simulink model "AFDNFSmodelSPA"  (R2017b)
settings: Solver=ode45  StartTime=0.0  StopTime=1400  FixedStep=1e-3  RelTol=1e-8  EnableMultiTasking=on
PostLoadFcn:
  | run('Methods/NFSOnLoad');
InitFcn:
  | run('Methods/AFDSimInit')
StopFcn:
  | run('Methods/NFSOnLoad');
values from neighbouring files (symbols this model uses):
  nfs = TransferFunction('Plot','true')    [Main.m]    (also in NFSDatabase.sldd = SI
                Imperial
                28184.4409185639)
undefined symbols (not defined in the file or in its folder): Continuous, desired, Earth, F, K_lat, K_long, Kobsvlat, Kobsvlong, lat, latsys, Light, long, longsys, MIL, Newton, Raphson, sigbuilder_block, Time, WGS84
libraries: simulink x6, aerolibtransform2 x2, aerolibwind2 x2, ModelsLibrary x1, ctrlSharedLib x1, sharedutil x1
(part 3 of 4)

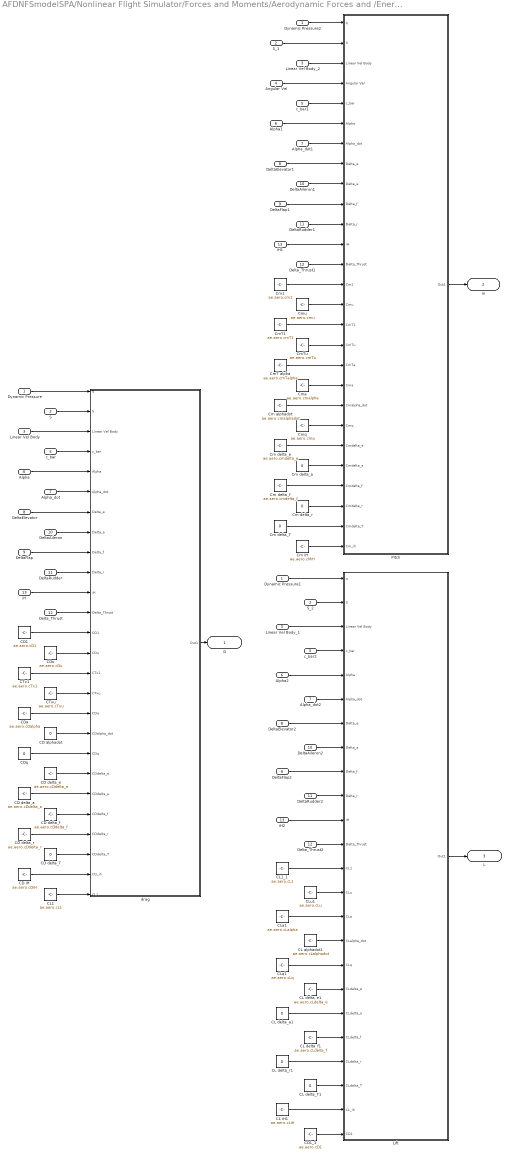
== system AFDNFSmodelSPA/Nonlinear Flight Simulator/Forces and Moments/Aerodynamic Forces and /Energy Analysis1/Longitudinal1 ==
  Dynamic Pressure : Inport
  S : Inport  Port=2
  Linear Vel Body : Inport  Port=3
  Angular Vel : Inport  Port=4
  c_bar : Inport  Port=5
  Alpha : Inport  Port=6
  Alpha_dot : Inport  Port=7
  DeltaElevator : Inport  Port=8
  DeltaFlap : Inport  Port=9
  DeltaAileron : Inport  Port=10
  DeltaRudder : Inport  Port=11
  Delta_Thrust : Inport  Port=12
  iH : Inport  Port=13
  Alpha1 : InportShadow  Port=6
  Alpha2 : InportShadow  Port=6
  Alpha_dot1 : InportShadow  Port=7
  Alpha_dot2 : InportShadow  Port=7
  CD alphadot : Constant  Value=0
  CD delta_T : Constant  Value=0
  CD delta_a : Constant  Value=ae.aero.cDdelta_a
  CD delta_e : Constant  Value=ae.aero.cDdelta_e
  CD delta_f : Constant  Value=ae.aero.cDdelta_f
  CD delta_r : Constant  Value=ae.aero.cDdelta_r
  CD iH : Constant  Value=ae.aero.cDiH
  CD1 : Constant  Value=ae.aero.cD1
  CD1_1 : Constant  Value=ae.aero.cD1
  CDa : Constant  Value=ae.aero.cDalpha
  CDq : Constant  Value=0
  CDu : Constant  Value=ae.aero.cDu
  CL alphadot1 : Constant  Value=ae.aero.cLalphadot
  CL delta_T1 : Constant  Value=0
  CL delta_a1 : Constant  Value=0
  CL delta_e1 : Constant  Value=ae.aero.cLdelta_e
  CL delta_f1 : Constant  Value=ae.aero.cLdelta_f
  CL delta_r1 : Constant  Value=0
  CL iH1 : Constant  Value=ae.aero.cLiH
  CL1 : Constant  Value=ae.aero.cL1
  CL1_1 : Constant  Value=ae.aero.cL1
  CLa1 : Constant  Value=ae.aero.cLalpha
  CLq1 : Constant  Value=ae.aero.cLq
  CLu1 : Constant  Value=ae.aero.cLu
  CTx1 : Constant  Value=ae.aero.cTx1
  CTxu : Constant  Value=ae.aero.cTxu
  Cm alphadot : Constant  Value=ae.aero.cmalphadot
  Cm delta_T : Constant  Value=0
  Cm delta_a : Constant  Value=0
  Cm delta_e : Constant  Value=ae.aero.cmdelta_e
  Cm delta_f : Constant  Value=ae.aero.cmdelta_f
  Cm delta_r : Constant  Value=0
  Cm iH : Constant  Value=ae.aero.cMiH
  Cm1 : Constant  Value=ae.aero.cm1
  CmT alpha : Constant  Value=ae.aero.cmTalpha
  CmT1 : Constant  Value=ae.aero.cmT1
  CmTu : Constant  Value=ae.aero.cmTu
  Cma : Constant  Value=ae.aero.cmalpha
  Cmq : Constant  Value=ae.aero.cmq
  Cmu : Constant  Value=ae.aero.cmu
  DeltaAileron1 : InportShadow  Port=10
  DeltaAileron2 : InportShadow  Port=10
  DeltaElevator1 : InportShadow  Port=8
  DeltaElevator2 : InportShadow  Port=8
  DeltaFlap1 : InportShadow  Port=9
  DeltaFlap2 : InportShadow  Port=9
  DeltaRudder1 : InportShadow  Port=11
  DeltaRudder2 : InportShadow  Port=11
  Delta_Thrust1 : InportShadow  Port=12
  Delta_Thrust2 : InportShadow  Port=12
  Dynamic Pressure1 : InportShadow
  Dynamic Pressure2 : InportShadow
  Lift : Subsystem
  Linear Vel Body_1 : InportShadow  Port=3
  Linear Vel Body_2 : InportShadow  Port=3
  Pitch : Subsystem
  S_1 : InportShadow  Port=2
  S_2 : InportShadow  Port=2
  c_bar1 : InportShadow  Port=5
  c_bar2 : InportShadow  Port=5
  drag : Subsystem
  iH1 : InportShadow  Port=13
  iH2 : InportShadow  Port=13
  D : Outport
  m : Outport  Port=2
  L : Outport  Port=3
  wires:
  DeltaRudder/1 -> drag/10(Delta_r)
  DeltaAileron/1 -> drag/8(Delta_a)
  CDa/1 -> drag/17(CDa)
  Alpha/1 -> drag/5(Alpha)
  CDu/1 -> drag/14(CDu)
  Alpha_dot/1 -> drag/6(Alpha_dot)
  drag/1(Out1) -> D/1
  Lift/1(Out1) -> L/1
  S/1 -> drag/2(S)
  Dynamic Pressure/1 -> drag/1(q)
  Linear Vel Body/1 -> drag/3(Linear Vel Body)
  Delta_Thrust/1 -> drag/12(Delta_Thrust)
  iH/1 -> drag/11(iH)
  CD delta_T/1 -> drag/24(CDdelta_T)
  DeltaElevator/1 -> drag/7(Delta_e)
  DeltaFlap/1 -> drag/9(Delta_f)
  Pitch/1(Out1) -> m/1
  c_bar/1 -> drag/4(c_bar)
  CD alphadot/1 -> drag/18(CDalpha_dot)
  CDq/1 -> drag/19(CDq)
  CD delta_e/1 -> drag/20(CDdelta_e)
  CD delta_a/1 -> drag/21(CDdelta_a)
  CD delta_f/1 -> drag/22(CDdelta_f)
  CD delta_r/1 -> drag/23(CDdelta_r)
  CD iH/1 -> drag/25(CD_ih)
  CTx1/1 -> drag/15(CTx1)
  CD1/1 -> drag/13(CD1)
  CTxu/1 -> drag/16(CTxu)
  DeltaRudder1/1 -> Pitch/11(Delta_r)
  DeltaAileron1/1 -> Pitch/9(Delta_a)
  Alpha1/1 -> Pitch/6(Alpha)
  Alpha_dot1/1 -> Pitch/7(Alpha_dot)
  S_1/1 -> Pitch/2(S)
  Dynamic Pressure2/1 -> Pitch/1(q)
  Linear Vel Body_2/1 -> Pitch/3(Linear Vel Body)
  Delta_Thrust1/1 -> Pitch/13(Delta_Thrust)
  iH1/1 -> Pitch/12(iH)
  DeltaElevator1/1 -> Pitch/8(Delta_e)
  DeltaFlap1/1 -> Pitch/10(Delta_f)
  S_2/1 -> Lift/2(S)
  Dynamic Pressure1/1 -> Lift/1(q)
  Linear Vel Body_1/1 -> Lift/3(Linear Vel Body)
  Delta_Thrust2/1 -> Lift/12(Delta_Thrust)
  c_bar2/1 -> Lift/4(c_bar)
  CL1/1 -> drag/26(CL1)
  iH2/1 -> Lift/11(iH)
  DeltaRudder2/1 -> Lift/10(Delta_r)
  DeltaFlap2/1 -> Lift/9(Delta_f)
  DeltaAileron2/1 -> Lift/8(Delta_a)
  DeltaElevator2/1 -> Lift/7(Delta_e)
  Alpha_dot2/1 -> Lift/6(Alpha_dot)
  Alpha2/1 -> Lift/5(Alpha)
  Angular Vel/1 -> Pitch/4(Angular Vel)
  c_bar1/1 -> Pitch/5(c_bar)
  CD1_1/1 -> Lift/24(CD1)
  CLa1/1 -> Lift/15(CLa)
  CLq1/1 -> Lift/17(CLq)
  CL delta_a1/1 -> Lift/19(CLdelta_a)
  CL delta_r1/1 -> Lift/21(CLdelta_r)
  CL iH1/1 -> Lift/23(CL_ih)
  CL delta_T1/1 -> Lift/22(CLdelta_T)
  CLu1/1 -> Lift/14(CLu)
  CL alphadot1/1 -> Lift/16(CLalpha_dot)
  CL delta_f1/1 -> Lift/20(CLdelta_f)
  CL delta_e1/1 -> Lift/18(CLdelta_e)
  CL1_1/1 -> Lift/13(CL1)
  CmT alpha/1 -> Pitch/18(CmTa)
  Cm alphadot/1 -> Pitch/20(Cmalpha_dot)
  Cm delta_e/1 -> Pitch/22(Cmdelta_e)
  Cm delta_f/1 -> Pitch/24(Cmdelta_f)
  Cm delta_T/1 -> Pitch/26(Cmdelta_T)
  CmT1/1 -> Pitch/16(CmT1)
  Cm1/1 -> Pitch/14(Cm1)
  CmTu/1 -> Pitch/17(CmTu)
  Cmq/1 -> Pitch/21(Cmq)
  Cm delta_a/1 -> Pitch/23(Cmdelta_a)
  Cm delta_r/1 -> Pitch/25(Cmdelta_r)
  Cmu/1 -> Pitch/15(Cmu)
  Cma/1 -> Pitch/19(Cma)
  Cm iH/1 -> Pitch/27(Cm_ih)

== system AFDNFSmodelSPA/Nonlinear Flight Simulator/Forces and Moments/Aerodynamic Forces and /Forces/Aerodynamic Forces ==
  note: Since the forces and moments are in stability axis,
      | the beta has been multiplied with zero.
  CL : Inport  PortDimensions=1
  CD : Inport  Port=2  PortDimensions=1
  CY : Inport  Port=3  PortDimensions=1
  Dynamic Pressure : Inport  Port=4  PortDimensions=1
  Alpha : Inport  Port=5  PortDimensions=1
  Beta : Inport  Port=6  PortDimensions=1
  ChSign : Gain  Gain=-1  SaturateOnIntegerOverflow=on  OutDataTypeStr=Inherit: Same as input  ParamDataTypeStr=Inherit: Same as input
  ChSign1 : Gain  Gain=-1  SaturateOnIntegerOverflow=on  OutDataTypeStr=Inherit: Same as input  ParamDataTypeStr=Inherit: Same as input
  ChSign2 : Gain  Gain=0  SaturateOnIntegerOverflow=on  OutDataTypeStr=Inherit: Same as input  ParamDataTypeStr=Inherit: Same as input
  Mux : Mux  Inputs=3
  Product{,2..4} (4 alike) : Product  SaturateOnIntegerOverflow=on  InputSameDT=on  OutDataTypeStr=Inherit: Same as first input
  Product1 : Product  Multiplication=Matrix(*)  SaturateOnIntegerOverflow=on  InputSameDT=on  OutDataTypeStr=Inherit: Same as first input
  Wind2Body TM : Subsystem
  Wing Area : Constant  Value=nfs.refarea
  Aerodynamic Forces : Outport  PortDimensions=[3,1]
  wires:
  Wind2Body TM/1(T_BW) -> Product1/1
  Product1/1 -> Aerodynamic Forces/1
  Beta/1 -> ChSign2/1
  CD/1 -> ChSign/1
  CL/1 -> ChSign1/1
  Alpha/1 -> Wind2Body TM/1(Alpha)
  Dynamic Pressure/1 -> Product/1
  Wing Area/1 -> Product/2
  Product/1 -> Product2/1, Product3/1, Product4/1
  ChSign/1 -> Product2/2
  CY/1 -> Product3/2
  ChSign1/1 -> Product4/2
  Product2/1 -> Mux/1
  Product3/1 -> Mux/2
  Product4/1 -> Mux/3
  Mux/1 -> Product1/2
  ChSign2/1 -> Wind2Body TM/2(Beta)

== system AFDNFSmodelSPA/Nonlinear Flight Simulator/Forces and Moments/Aerodynamic Forces and /Forces/Force Coefficients Calculator ==
  Linear Velocity : Inport  PortDimensions=[3,1]
  Alpha : Inport  Port=2  PortDimensions=1
  Beta : Inport  Port=3
  Angular Velocity : Inport  Port=4  PortDimensions=[3,1]
  Control : Inport  Port=5  PortDimensions=[4,1]
  Alphadot : Inport  Port=6  PortDimensions=1
  Mach : Inport  Port=7
  Alpha2 : InportShadow  Port=2  PortDimensions=1
  Angular Velocity1 : InportShadow  Port=4  PortDimensions=[3,1]
  Control1 : InportShadow  Port=5  PortDimensions=[4,1]
  Demux1 : Demux  Outputs=3
  Demux2 : Demux  Outputs=3
  Demux3 : Demux
  Demux4 : Demux
  Drag Coefficient : Subsystem  mask{cD0=nfs.aero.cD0}
  Lift Coefficient : Subsystem  mask{cL0=nfs.aero.cL0, meanchord=nfs.meanchord}
      mask prompts: meanchord "Mean Aerodynamic Chord"
  Linear Velocity1 : InportShadow  PortDimensions=[3,1]
  Mach1 : InportShadow  Port=7
  SideForce Coefficient : Subsystem
  Terminator{,1..4} (5 alike) : Terminator
  CL : Outport
  CD : Outport  Port=2
  CY : Outport  Port=3
  wires:
  Linear Velocity/1 -> Lift Coefficient/1(Linear Velocity)
  SideForce Coefficient/1(CY) -> CY/1
  Drag Coefficient/1(CD) -> CD/1
  Alpha2/1 -> Drag Coefficient/2(alpha)
  Demux1/3 -> Terminator1/1
  Alphadot/1 -> Lift Coefficient/5(Alphadot)
  Lift Coefficient/1(CL) -> CL/1, Drag Coefficient/1(CL)
  Demux2/1 -> SideForce Coefficient/3(P)
  Demux3/1 -> Lift Coefficient/3(DeltaElevator)
  Control1/1 -> Demux4/1
  Demux2/3 -> SideForce Coefficient/4(R)
  Angular Velocity1/1 -> Demux2/1
  Beta/1 -> SideForce Coefficient/2(Beta)
  Demux1/1 -> Terminator/1
  Control/1 -> Demux3/1
  Angular Velocity/1 -> Demux1/1
  Demux4/2 -> Drag Coefficient/4(DeltaFlap)
  Mach/1 -> Lift Coefficient/7(Mach)
  Demux1/2 -> Lift Coefficient/6(Q)
  Demux3/4 -> Terminator4/1
  Demux3/3 -> Terminator3/1
  Alpha/1 -> Lift Coefficient/2(Alpha)
  Demux2/2 -> Terminator2/1
  Demux4/4 -> SideForce Coefficient/6(DeltaRudder), Drag Coefficient/6(DeltaRudder)
  Demux4/3 -> SideForce Coefficient/5(DeltaAileron), Drag Coefficient/5(DeltaAileron)
  Demux4/1 -> Drag Coefficient/3(DeltaElevator)
  Mach1/1 -> Drag Coefficient/7(Mach)
  Demux3/2 -> Lift Coefficient/4(DeltaFlap)
  Linear Velocity1/1 -> SideForce Coefficient/1(Linear Velocity)

== system AFDNFSmodelSPA/Nonlinear Flight Simulator/Forces and Moments/Aerodynamic Forces and /Moments/Aerodynamic Moment  ==
  note: Since the forces and moments are in stability axis,
      | the beta has been multiplied with zero.
  Cl : Inport
  Cm : Inport  Port=2
  Cn : Inport  Port=3
  Dynamic Pressure : Inport  Port=4
  Alpha : Inport  Port=5  PortDimensions=1
  Beta : Inport  Port=6  PortDimensions=1
  Dynamic Pressure1 : InportShadow  Port=4
  Dynamic Pressure2 : InportShadow  Port=4
  Gain : Gain  Gain=0
  Mux : Mux  Inputs=3
  Pitch : Product  Inputs=4  SaturateOnIntegerOverflow=on  InputSameDT=on  OutDataTypeStr=Inherit: Same as first input
  Product1 : Product  Multiplication=Matrix(*)  SaturateOnIntegerOverflow=on  InputSameDT=on  OutDataTypeStr=Inherit: Same as first input
  Roll : Product  Inputs=4  SaturateOnIntegerOverflow=on  InputSameDT=on  OutDataTypeStr=Inherit: Same as first input
  Wind2Body TM : Subsystem
  Wing area : Constant  Value=nfs.refarea
  Wing chord : Constant  Value=nfs.meanchord
  Wing span : Constant  Value=nfs.span
  Wing span2 : Constant  Value=nfs.span
  Yaw : Product  Inputs=4  SaturateOnIntegerOverflow=on  InputSameDT=on  OutDataTypeStr=Inherit: Same as first input
  Aerodynamic Moments : Outport  PortDimensions=[3,1]
  wires:
  Yaw/1 -> Mux/3
  Pitch/1 -> Mux/2
  Roll/1 -> Mux/1
  Wing area/1 -> Yaw/2, Roll/2, Pitch/2
  Wing span2/1 -> Yaw/3
  Dynamic Pressure2/1 -> Yaw/1
  Dynamic Pressure1/1 -> Pitch/1
  Cl/1 -> Roll/4
  Cm/1 -> Pitch/4
  Cn/1 -> Yaw/4
  Dynamic Pressure/1 -> Roll/1
  Wing chord/1 -> Pitch/3
  Wing span/1 -> Roll/3
  Wind2Body TM/1(T_BW) -> Product1/1
  Beta/1 -> Gain/1
  Alpha/1 -> Wind2Body TM/1(Alpha)
  Mux/1 -> Product1/2
  Product1/1 -> Aerodynamic Moments/1
  Gain/1 -> Wind2Body TM/2(Beta)

== system AFDNFSmodelSPA/Nonlinear Flight Simulator/Forces and Moments/Aerodynamic Forces and /Moments/Pitch Moment Coefficient ==
  Linear Velocity : Inport
  Alpha : Inport  Port=2
  Q : Inport  Port=3
  DeltaElevator : Inport  Port=4
  DeltaFlap : Inport  Port=5
  Alphadot : Inport  Port=6  PortDimensions=1
  Mach : Inport  Port=7  PortDimensions=1
  2 : Gain  Gain=2  SaturateOnIntegerOverflow=on  OutDataTypeStr=Inherit: Same as input  ParamDataTypeStr=Inherit: Same as input
  Cm*c/(2V) : Product  Inputs=**/  SaturateOnIntegerOverflow=on  InputSameDT=on  OutDataTypeStr=Inherit: Same as first input
  Cm0 : Constant  Value=nfs.aero.cm0
  Scope{1..7} (7 alike) : Scope
  Sum : Sum  SaturateOnIntegerOverflow=on  InputSameDT=on  OutDataTypeStr=Inherit: Same as first input
  Sum2 : Sum  Inputs=++++++  SaturateOnIntegerOverflow=on  InputSameDT=on  OutDataTypeStr=Inherit: Same as first input
  Velocity Magnitude : Subsystem
  Wing chord : Constant  Value=nfs.meanchord
  cmM : Gain  Gain=nfs.aero.cmM  SaturateOnIntegerOverflow=on  OutDataTypeStr=Inherit: Same as input  ParamDataTypeStr=Inherit: Same as input
  cmalpha : Gain  Gain=nfs.aero.cmalpha  SaturateOnIntegerOverflow=on  OutDataTypeStr=Inherit: Same as input  ParamDataTypeStr=Inherit: Same as input
  cmalphadot : Gain  Gain=nfs.aero.cmalphadot  SaturateOnIntegerOverflow=on  OutDataTypeStr=Inherit: Same as input  ParamDataTypeStr=Inherit: Same as input
  cmdelta_e : Gain  Gain=nfs.aero.cmdelta_e  SaturateOnIntegerOverflow=on  OutDataTypeStr=Inherit: Same as input  ParamDataTypeStr=Inherit: Same as input
  cmdelta_f : Gain  Gain=nfs.aero.cmdelta_f  SaturateOnIntegerOverflow=on  OutDataTypeStr=Inherit: Same as input  ParamDataTypeStr=Inherit: Same as input
  cmq : Gain  Gain=nfs.aero.cmq  SaturateOnIntegerOverflow=on  OutDataTypeStr=Inherit: Same as input  ParamDataTypeStr=Inherit: Same as input
  Cm : Outport  PortDimensions=1
  wires:
  Sum2/1 -> Cm/1
  Mach/1 -> cmM/1
  Q/1 -> cmq/1
  DeltaElevator/1 -> cmdelta_e/1
  DeltaFlap/1 -> cmdelta_f/1
  Alpha/1 -> cmalpha/1
  Velocity Magnitude/1(Velocity Magnitude) -> 2/1
  Linear Velocity/1 -> Velocity Magnitude/1(Velocity)
  cmM/1 -> Sum2/6, Scope6/1
  Cm*c/(2V)/1 -> Sum2/5
  cmdelta_e/1 -> Sum2/4, Scope3/1
  cmdelta_f/1 -> Sum2/3, Scope2/1
  cmalpha/1 -> Sum2/2, Scope1/1
  Cm0/1 -> Sum2/1, Scope7/1
  Sum/1 -> Cm*c/(2V)/1
  cmalphadot/1 -> Sum/1, Scope4/1
  cmq/1 -> Sum/2, Scope5/1
  Wing chord/1 -> Cm*c/(2V)/2
  2/1 -> Cm*c/(2V)/3
  Alphadot/1 -> cmalphadot/1

== system AFDNFSmodelSPA/Nonlinear Flight Simulator/Forces and Moments/Aerodynamic Forces and /Moments/Roll Moment Coefficient ==
  Linear Velocity : Inport
  Beta : Inport  Port=2  PortDimensions=1
  P : Inport  Port=3
  R : Inport  Port=4
  DeltaAileron : Inport  Port=5
  DeltaRudder : Inport  Port=6
  2 : Gain  Gain=2  SaturateOnIntegerOverflow=on  OutDataTypeStr=Inherit: Same as input  ParamDataTypeStr=Inherit: Same as input
  Cl*b/(2V) : Product  Inputs=**/  SaturateOnIntegerOverflow=on  InputSameDT=on  OutDataTypeStr=Inherit: Same as first input
  Sum : Sum  SaturateOnIntegerOverflow=on  InputSameDT=on  OutDataTypeStr=Inherit: Same as first input
  Sum2 : Sum  Inputs=++++  SaturateOnIntegerOverflow=on  InputSameDT=on  OutDataTypeStr=Inherit: Same as first input
  Velocity Magnitude : Subsystem
  Wing span : Constant  Value=nfs.span
  clbeta : Gain  Gain=nfs.aero.clbeta  SaturateOnIntegerOverflow=on  OutDataTypeStr=Inherit: Same as input  ParamDataTypeStr=Inherit: Same as input
  cldelta_a : Gain  Gain=nfs.aero.cldelta_a  SaturateOnIntegerOverflow=on  OutDataTypeStr=Inherit: Same as input  ParamDataTypeStr=Inherit: Same as input
  cldelta_r : Gain  Gain=nfs.aero.cldelta_r  SaturateOnIntegerOverflow=on  OutDataTypeStr=Inherit: Same as input  ParamDataTypeStr=Inherit: Same as input
  clp : Gain  Gain=nfs.aero.clp  SaturateOnIntegerOverflow=on  OutDataTypeStr=Inherit: Same as input  ParamDataTypeStr=Inherit: Same as input
  clr : Gain  Gain=nfs.aero.clr  SaturateOnIntegerOverflow=on  OutDataTypeStr=Inherit: Same as input  ParamDataTypeStr=Inherit: Same as input
  Cl : Outport  PortDimensions=1
  wires:
  Sum2/1 -> Cl/1
  R/1 -> clr/1
  P/1 -> clp/1
  DeltaRudder/1 -> cldelta_r/1
  DeltaAileron/1 -> cldelta_a/1
  Beta/1 -> clbeta/1
  Velocity Magnitude/1(Velocity Magnitude) -> 2/1
  Linear Velocity/1 -> Velocity Magnitude/1(Velocity)
  Cl*b/(2V)/1 -> Sum2/4
  cldelta_r/1 -> Sum2/3
  cldelta_a/1 -> Sum2/2
  clbeta/1 -> Sum2/1
  2/1 -> Cl*b/(2V)/3
  Wing span/1 -> Cl*b/(2V)/2
  Sum/1 -> Cl*b/(2V)/1
  clr/1 -> Sum/2
  clp/1 -> Sum/1

== system AFDNFSmodelSPA/Nonlinear Flight Simulator/Forces and Moments/Aerodynamic Forces and /Moments/Yaw Moment Coefficient ==
  Linear Velocity : Inport
  beta : Inport  Port=2  PortDimensions=1
  P : Inport  Port=3
  R : Inport  Port=4
  DeltaAileron : Inport  Port=5
  DeltaRudder : Inport  Port=6
  2 : Gain  Gain=2  SaturateOnIntegerOverflow=on  OutDataTypeStr=Inherit: Same as input  ParamDataTypeStr=Inherit: Same as input
  Cn*b/(2V) : Product  Inputs=**/  SaturateOnIntegerOverflow=on  InputSameDT=on  OutDataTypeStr=Inherit: Same as first input
  Sum : Sum  SaturateOnIntegerOverflow=on  InputSameDT=on  OutDataTypeStr=Inherit: Same as first input
  Sum2 : Sum  Inputs=++++  SaturateOnIntegerOverflow=on  InputSameDT=on  OutDataTypeStr=Inherit: Same as first input
  Velocity Magnitude : Subsystem
  Wing span : Constant  Value=nfs.span
  cnbeta : Gain  Gain=nfs.aero.cnbeta  SaturateOnIntegerOverflow=on  OutDataTypeStr=Inherit: Same as input  ParamDataTypeStr=Inherit: Same as input
  cndelta_a : Gain  Gain=nfs.aero.cndelta_a  SaturateOnIntegerOverflow=on  OutDataTypeStr=Inherit: Same as input  ParamDataTypeStr=Inherit: Same as input
  cndelta_r : Gain  Gain=nfs.aero.cndelta_r  SaturateOnIntegerOverflow=on  OutDataTypeStr=Inherit: Same as input  ParamDataTypeStr=Inherit: Same as input
  cnp : Gain  Gain=nfs.aero.cnp  SaturateOnIntegerOverflow=on  OutDataTypeStr=Inherit: Same as input  ParamDataTypeStr=Inherit: Same as input
  cnr : Gain  Gain=nfs.aero.cnr  SaturateOnIntegerOverflow=on  OutDataTypeStr=Inherit: Same as input  ParamDataTypeStr=Inherit: Same as input
  Cn : Outport  PortDimensions=1
  wires:
  Sum2/1 -> Cn/1
  R/1 -> cnr/1
  P/1 -> cnp/1
  DeltaRudder/1 -> cndelta_r/1
  DeltaAileron/1 -> cndelta_a/1
  beta/1 -> cnbeta/1
  Velocity Magnitude/1(Velocity Magnitude) -> 2/1
  Linear Velocity/1 -> Velocity Magnitude/1(Velocity)
  cnp/1 -> Sum/1
  cnr/1 -> Sum/2
  Sum/1 -> Cn*b/(2V)/1
  Wing span/1 -> Cn*b/(2V)/2
  2/1 -> Cn*b/(2V)/3
  cnbeta/1 -> Sum2/1
  cndelta_a/1 -> Sum2/2
  cndelta_r/1 -> Sum2/3
  Cn*b/(2V)/1 -> Sum2/4

== system AFDNFSmodelSPA/Nonlinear Flight Simulator/Forces and Moments/Aerodynamic Forces and /Turbulence/Turbulence Model ==
  In : Inport
  Dryden Turbulence Model : Subsystem  VariantControl=TurbulenceSelector == 1
  No Turbulence : Subsystem  VariantControl=TurbulenceSelector == 0
  Von-Karman Turbulence Model : Subsystem  VariantControl=TurbulenceSelector == 2
  Out : Outport

== system AFDNFSmodelSPA/OnBoardComputer/Control System/Trim Offset + Reference Excitation/Doublet Generated Signal/Doublet ==
  Step : Step  Time=T_start  After=amp  SampleTime=sampletime
  Step1 : Step  Time=T_start+span/2  After=amp  SampleTime=sampletime
  Step2 : Step  Time=T_start+span/2  After=-amp  SampleTime=sampletime
  Step3 : Step  Time=T_start+span  After=-amp  SampleTime=sampletime
  Sum : Sum  Inputs=|+-
  Sum1 : Sum  Inputs=|+-
  Sum2 : Sum  Inputs=|++
  Out1 : Outport
  wires:
  Step/1 -> Sum/1
  Step1/1 -> Sum/2
  Step2/1 -> Sum1/1
  Step3/1 -> Sum1/2
  Sum/1 -> Sum2/1
  Sum1/1 -> Sum2/2
  Sum2/1 -> Out1/1

== system AFDNFSmodelSPA/OnBoardComputer/Control System/Trim Offset + Reference Excitation/Triangular signal span 10 sec/Signal Builder1 ==
  Demux : Demux  Tag=STV Demux  Outputs=1
  FromWs : FromWorkspace  Tag=STV FromWs  VariableName=tuvar  SampleTime=0
      SigBuilderData=|
      | common.afterFinalStr = 'Extrapolate'
      | common.sampleTime = 0
      | dataSet.timeRange = [10 20]
      | dataSet.name = 'Group 1'
      | sbobj.Groups.Name = 'Group 1'
      | sbobj.Groups.Signals.Name = 'Normalized Elevator(deg)'
      | sbobj.Groups.Signals.XData = [10 11 12 13 14 15 16 17 20]
      | sbobj.Groups.Signals.YData = [0 0 0.25 0 -0.25 0 0 0 0]
      | sbobj.Groups.TimeRange = [10 20]
  Normalized Elevator(deg) : Outport  Tag=STV Outport
  wires:
  FromWs/1 -> Demux/1
  Demux/1 -> Normalized Elevator(deg)/1

== system AFDNFSmodelSPA/OnBoardComputer/Control System/Trim Offset + Reference Excitation/Triangular signal span 10 sec/Signal Builder2 ==
  Demux : Demux  Tag=STV Demux  Outputs=1
  FromWs : FromWorkspace  Tag=STV FromWs  VariableName=tuvar  SampleTime=0
      SigBuilderData=|
      | common.afterFinalStr = 'Extrapolate'
      | common.sampleTime = 0
      | dataSet.timeRange = [10 20]
      | dataSet.name = 'Group 1'
      | sbobj.Groups.Name = 'Group 1'
      | sbobj.Groups.Signals.Name = 'Normalized Flap(deg)'
      | sbobj.Groups.Signals.XData = [10 11 12 13 14 15 16 17 20]
      | sbobj.Groups.Signals.YData = [0 0 0 0 0 0 0 0 0]
      | sbobj.Groups.TimeRange = [10 20]
  Normalized Flap(deg) : Outport  Tag=STV Outport
  wires:
  Demux/1 -> Normalized Flap(deg)/1
  FromWs/1 -> Demux/1

== system AFDNFSmodelSPA/OnBoardComputer/Control System/Trim Offset + Reference Excitation/Triangular signal span 10 sec/Signal Builder3 ==
  Demux : Demux  Tag=STV Demux  Outputs=1
  FromWs : FromWorkspace  Tag=STV FromWs  VariableName=tuvar  SampleTime=0
      SigBuilderData=|
      | common.afterFinalStr = 'Extrapolate'
      | common.sampleTime = 0
      | dataSet.timeRange = [10 20]
      | dataSet.name = 'Group 1'
      | sbobj.Groups.Name = 'Group 1'
      | sbobj.Groups.Signals.Name = 'Normalized Alileron(deg)'
      | sbobj.Groups.Signals.XData = [10 11 12 13 14 15 16 17 20]
      | sbobj.Groups.Signals.YData = [0 0 0.1 0 -0.1 0 0 0 0]
      | sbobj.Groups.TimeRange = [10 20]
  Normalized Alileron(deg) : Outport  Tag=STV Outport
  wires:
  FromWs/1 -> Demux/1
  Demux/1 -> Normalized Alileron(deg)/1

== system AFDNFSmodelSPA/OnBoardComputer/Control System/Trim Offset + Reference Excitation/Triangular signal span 10 sec/Signal Builder4 ==
  Demux : Demux  Tag=STV Demux  Outputs=1
  FromWs : FromWorkspace  Tag=STV FromWs  VariableName=tuvar  SampleTime=0
      SigBuilderData=|
      | common.afterFinalStr = 'Extrapolate'
      | common.sampleTime = 0
      | dataSet.timeRange = [10 20]
      | dataSet.name = 'Group 1'
      | sbobj.Groups.Name = 'Group 1'
      | sbobj.Groups.Signals.Name = 'Normalized Rudder(deg)'
      | sbobj.Groups.Signals.XData = [10 11 12 13 14 15 16 17 20]
      | sbobj.Groups.Signals.YData = [0 0 0.6 0 -0.6 0 0 0 0]
      | sbobj.Groups.TimeRange = [10 20]
  Normalized Rudder(deg) : Outport  Tag=STV Outport
  wires:
  Demux/1 -> Normalized Rudder(deg)/1
  FromWs/1 -> Demux/1

== system AFDNFSmodelSPA/Navigation & Sensor System/Navigation Model/01-Test Model/Navigation Model - Simple/Euler angles & Direction Cosine Using Quaternions/If Action Subsystem ==
  Simulation Termination : Inport
  Action Port : ActionPort
  Stop Simulation : Stop
  wires:
  Simulation Termination/1 -> Stop Simulation/1

== system AFDNFSmodelSPA/Navigation & Sensor System/Navigation Model/01-Test Model/Navigation Model - Simple/Euler angles & Direction Cosine Using Quaternions/Quaternion Rates ==
  Angular Velocities : Inport  PortDimensions=[3,1]
  Quaternions : Inport  Port=2  PortDimensions=4
  Constant : Constant
  Dot Product : DotProduct  OutDataTypeStr=Inherit: Inherit via internal rule
  High Gain Quaternion Normalization : Gain  Gain=10  SaturateOnIntegerOverflow=on  OutDataTypeStr=Inherit: Same as input  ParamDataTypeStr=Inherit: Same as input
  Mux3 : Mux  Inputs=[3 4 1]
  Mux4 : Mux
  Sum : Sum  Inputs=|+-  SaturateOnIntegerOverflow=on  InputSameDT=on  OutDataTypeStr=Inherit: Same as first input
  q0dot : Fcn  Expr=-0.5 * ( u[5]*u[1]+u[6]*u[2]+u[7]*u[3] ) + u[8]*u[4]
  q1dot : Fcn  Expr=0.5 * ( u[4]*u[1]+u[6]*u[3]-u[7]*u[2] ) + u[8]*u[5]
  q2dot : Fcn  Expr=0.5 * ( u[4]*u[2]+u[7]*u[1]-u[5]*u[3] ) + u[8]*u[6]
  q3dot : Fcn  Expr=0.5 * ( u[4]*u[3]+u[5]*u[2]-u[6]*u[1] ) + u[8]*u[7]
  Quaternion Rates : Outport  PortDimensions=4  InitialOutput=0
  wires:
  Angular Velocities/1 -> Mux3/1
  Dot Product/1 -> Sum/2
  High Gain Quaternion Normalization/1 -> Mux3/3
  Sum/1 -> High Gain Quaternion Normalization/1
  Constant/1 -> Sum/1
  Mux4/1 -> Quaternion Rates/1
  q0dot/1 -> Mux4/1
  q1dot/1 -> Mux4/2
  q2dot/1 -> Mux4/3
  Mux3/1 -> q2dot/1, q3dot/1, q0dot/1, q1dot/1
  q3dot/1 -> Mux4/4
  Quaternions/1 -> Dot Product/1, Dot Product/2, Mux3/2

== system AFDNFSmodelSPA/Navigation & Sensor System/Navigation Model/01-Test Model/Navigation Model - Simple/Euler angles & Direction Cosine Using Quaternions/Rotation Angles to DCM1 ==
  q : Inport  PortDimensions=4
  Create Transformation Matrix : Subsystem
  Quaternion Normalize : Subsystem
  a11 : Subsystem
  a12 : Subsystem
  a13 : Subsystem
  a21 : Subsystem
  a22 : Subsystem
  a23 : Subsystem
  a31 : Subsystem
  a32 : Subsystem
  a33 : Subsystem
  DCM : Outport  PortDimensions=[3,3]
  wires:
  q/1 -> Quaternion Normalize/1(q)
  a11/1(A11) -> Create Transformation Matrix/1(M11)
  a12/1(A12) -> Create Transformation Matrix/2(M12)
  a13/1(A13) -> Create Transformation Matrix/3(M13)
  a21/1(A21) -> Create Transformation Matrix/4(M21)
  a22/1(A22) -> Create Transformation Matrix/5(M22)
  a23/1(A23) -> Create Transformation Matrix/6(M23)
  a31/1(A31) -> Create Transformation Matrix/7(M31)
  a32/1(A32) -> Create Transformation Matrix/8(M32)
  a33/1(A33) -> Create Transformation Matrix/9(M33)
  Quaternion Normalize/1(normal(q)) -> a33/1(normal(q)), a32/1(normal(q)), a31/1(normal(q)), a23/1(normal(q)), a22/1(normal(q)), a21/1(normal(q)), a13/1(normal(q)), a12/1(normal(q)), a11/1(normal(q))
  Create Transformation Matrix/1(Matrix) -> DCM/1

== system AFDNFSmodelSPA/Navigation & Sensor System/Navigation Model/01-Test Model/Navigation Model - Simple/Euler angles & Direction Cosine Using Quaternions/Rotation Angles to Quaternions ==
  "[R1,R2,R3]" : Inport  PortDimensions=3
  1/2 : Gain  Gain=0.5  SaturateOnIntegerOverflow=on  OutDataTypeStr=Inherit: Same as input  ParamDataTypeStr=Inherit: Same as input
  Mux1 : Mux  Inputs=2
  Mux2 : Mux
  q0 : Fcn  Expr=u(4)*u(5)*u(6) + u(1)*u(2)*u(3)
  q1 : Fcn  Expr=u(4)*u(5)*u(3) - u(1)*u(2)*u(6)
  q2 : Fcn  Expr=u(4)*u(2)*u(6) + u(1)*u(5)*u(3)
  q3 : Fcn  Expr=u(1)*u(5)*u(6) - u(4)*u(2)*u(3)
  sincos : Trigonometry  Operator=sincos
  Quat : Outport  PortDimensions=4
  wires:
  q0/1 -> Mux2/1
  Mux2/1 -> Quat/1
  q3/1 -> Mux2/4
  q2/1 -> Mux2/3
  q1/1 -> Mux2/2
  Mux1/1 -> q3/1, q2/1, q1/1, q0/1
  sincos/2 -> Mux1/2
  sincos/1 -> Mux1/1
  1/2/1 -> sincos/1
  "[R1,R2,R3]"/1 -> 1/2/1

== system AFDNFSmodelSPA/Navigation & Sensor System/Navigation Model/01-Test Model/Navigation Model - Simple/Euler angles & Direction Cosine Using Quaternions/Rotation Angles to Quaternions1 ==
  q : Inport  PortDimensions=4
  Quaternion Normalize : Subsystem
  Trigonometric Function1 : Trigonometry  Operator=atan2
  Trigonometric Function3 : Trigonometry  Operator=atan2
  Vector Concatenate : Concatenate  NumInputs=3
  fcn1 : Fcn  Expr=2*(u[2]*u[3] + u[1]*u[4])
  fcn2 : Fcn  Expr=u[1]*u[1] + u[2]*u[2] - u[3]*u[3] - u[4]*u[4]
  fcn3 : Fcn  Expr=-2*(u[2]*u[4] - u[1]*u[3])
  fcn4 : Fcn  Expr=2*(u[3]*u[4] + u[1]*u[2])
  fcn5 : Fcn  Expr=u[1]*u[1] - u[2]*u[2] - u[3]*u[3] + u[4]*u[4]
  trigFcn : Trigonometry  Operator=asin
  Quat2RotAngs : Outport  PortDimensions=[3,1]
  wires:
  fcn5/1 -> Trigonometric Function3/2
  fcn4/1 -> Trigonometric Function3/1
  fcn2/1 -> Trigonometric Function1/2
  fcn1/1 -> Trigonometric Function1/1
  fcn3/1 -> trigFcn/1
  Trigonometric Function1/1 -> Vector Concatenate/1  "r1"
  trigFcn/1 -> Vector Concatenate/2  "r2"
  Trigonometric Function3/1 -> Vector Concatenate/3  "r3"
  Quaternion Normalize/1(normal(q)) -> fcn1/1, fcn2/1, fcn5/1, fcn4/1, fcn3/1
  q/1 -> Quaternion Normalize/1(q)
  Vector Concatenate/1 -> Quat2RotAngs/1

== system AFDNFSmodelSPA/Navigation & Sensor System/Navigation Model/01-Test Model/Navigation Model - Simple/Euler angles & Direction Cosine Using Quaternions/Transform from Body to Inertial axes ==
  Transformation Matrix : Inport
  Position Vector : Inport  Port=2
  Product : Product  Multiplication=Matrix(*)  SaturateOnIntegerOverflow=on  InputSameDT=on  OutDataTypeStr=Inherit: Same as first input
  Reshape1 : Reshape  OutputDimensionality=Column vector (2-D)
  Reshape2 : Reshape
  Ve : Outport
  wires:
  Product/1 -> Reshape2/1
  Transformation Matrix/1 -> Product/1
  Position Vector/1 -> Reshape1/1
  Reshape1/1 -> Product/2
  Reshape2/1 -> Ve/1

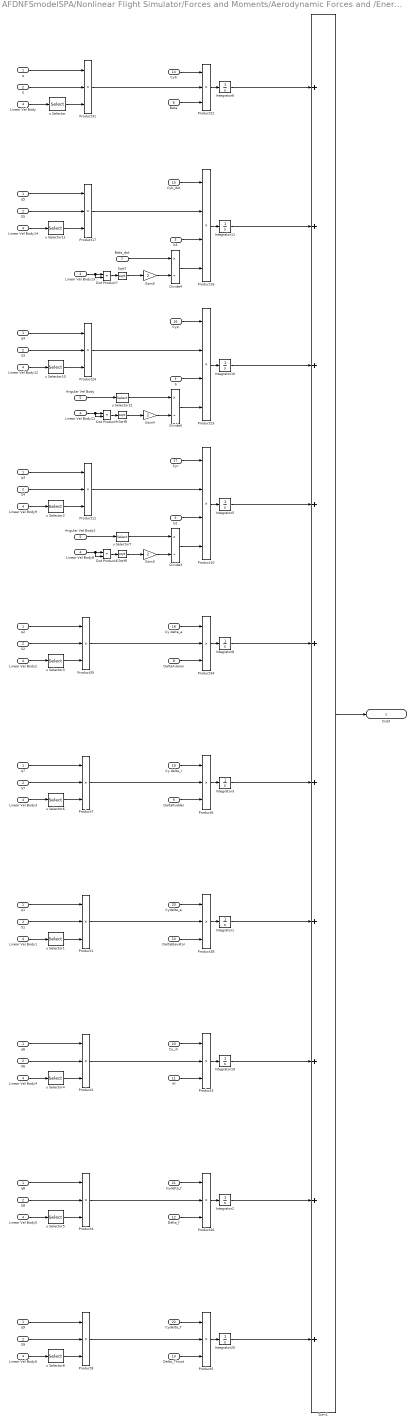
== system AFDNFSmodelSPA/Nonlinear Flight Simulator/Forces and Moments/Aerodynamic Forces and /Energy Analysis1/Lateral-Directional1/Fy ==
  q : Inport
  S : Inport  Port=2
  b : Inport  Port=3
  Linear Vel Body : Inport  Port=4
  Angular Vel Body : Inport  Port=5
  Beta : Inport  Port=6
  Beta_dot : Inport  Port=7
  DeltaAileron : Inport  Port=8
  DeltaRudder : Inport  Port=9
  DeltaElevator : Inport  Port=10
  iH : Inport  Port=11
  Delta_f : Inport  Port=12
  Delta_Thrust : Inport  Port=13
  Cyb : Inport  Port=14
  Cyb_dot : Inport  Port=15
  Cyp : Inport  Port=16
  Cyr : Inport  Port=17
  Cy delta_a : Inport  Port=18
  Cy delta_r : Inport  Port=19
  Cydelta_e : Inport  Port=20
  Cydelta_f : Inport  Port=21
  Cydelta_T : Inport  Port=22
  Cy_ih : Inport  Port=23
  Angular Vel Body2 : InportShadow  Port=5
  Divide3 : Product  Inputs=*/
  Divide4 : Product  Inputs=*/
  Divide5 : Product  Inputs=*/
  Dot Product6 : DotProduct  InputSameDT=on  OutDataTypeStr=Inherit: Inherit via internal rule
  Dot Product7 : DotProduct  InputSameDT=on  OutDataTypeStr=Inherit: Inherit via internal rule
  Dot Product9 : DotProduct  InputSameDT=on  OutDataTypeStr=Inherit: Inherit via internal rule
  Gain3 : Gain  Gain=2
  Gain4 : Gain  Gain=2
  Gain5 : Gain  Gain=2
  Integrator{1..3,5..6,8,10..11,19..20} (10 alike) : Integrator
  Linear Vel Body{1..6,8..9,11..14} (12 alike) : InportShadow  Port=4
  Product{1..8,11,17,22,24,26,28,31,34..35} (17 alike) : Product  Inputs=3
  Product10 : Product  Inputs=4
  Product16 : Product  Inputs=4
  Product23 : Product  Inputs=4
  S{1..9} (9 alike) : InportShadow  Port=2
  Sqrt6 : Sqrt  SaturateOnIntegerOverflow=on
  Sqrt7 : Sqrt  SaturateOnIntegerOverflow=on
  Sqrt8 : Sqrt  SaturateOnIntegerOverflow=on
  Sum1 : Sum  Inputs=++++++++++
  b2 : InportShadow  Port=3
  b3 : InportShadow  Port=3
  q{1..9} (9 alike) : InportShadow
  u Selector{,1..6,8,10..11} (10 alike) : Selector  InputPortWidth=3  IndexOptions=Index vector (dialog)  Indices=[2]  OutputSizes=1
  u Selector12 : Selector  InputPortWidth=3  IndexOptions=Index vector (dialog)  Indices=[1]  OutputSizes=1
  u Selector7 : Selector  InputPortWidth=3  IndexOptions=Index vector (dialog)  Indices=[3]  OutputSizes=1
  Out3 : Outport
  wires:
  Integrator11/1 -> Sum1/2
  q/1 -> Product31/1
  S/1 -> Product31/2
  u Selector/1 -> Product31/3
  Linear Vel Body/1 -> u Selector/1
  Cy delta_a/1 -> Product34/1
  Product35/1 -> Product34/2
  DeltaAileron/1 -> Product34/3
  Product34/1 -> Integrator8/1
  Integrator8/1 -> Sum1/5
  Product24/1 -> Product23/2
  Divide5/1 -> Product23/4
  Product23/1 -> Integrator10/1
  q4/1 -> Product24/1
  S3/1 -> Product24/2
  u Selector10/1 -> Product24/3
  Linear Vel Body12/1 -> u Selector10/1
  Sqrt8/1 -> Gain4/1
  u Selector12/1 -> Divide5/1
  Dot Product9/1 -> Sqrt8/1
  Linear Vel Body11/1 -> Dot Product9/2, Dot Product9/1
  Angular Vel Body/1 -> u Selector12/1
  Cyp/1 -> Product23/1
  Sum1/1 -> Out3/1
  Cyb/1 -> Product22/1
  Product31/1 -> Product22/2
  Beta/1 -> Product22/3
  Product22/1 -> Integrator6/1
  Integrator6/1 -> Sum1/1
  b/1 -> Product23/3
  Gain4/1 -> Divide5/2
  Product11/1 -> Product10/2
  Divide3/1 -> Product10/4
  Product10/1 -> Integrator5/1
  q3/1 -> Product11/1
  S4/1 -> Product11/2
  u Selector2/1 -> Product11/3
  Linear Vel Body9/1 -> u Selector2/1
  Sqrt6/1 -> Gain3/1
  u Selector7/1 -> Divide3/1
  Dot Product6/1 -> Sqrt6/1
  Linear Vel Body8/1 -> Dot Product6/1, Dot Product6/2
  Angular Vel Body2/1 -> u Selector7/1
  Cyr/1 -> Product10/1
  b2/1 -> Product10/3
  Gain3/1 -> Divide3/2
  Integrator10/1 -> Sum1/3
  Integrator5/1 -> Sum1/4
  Product17/1 -> Product16/2
  Divide4/1 -> Product16/4
  Product16/1 -> Integrator11/1
  q5/1 -> Product17/1
  S5/1 -> Product17/2
  u Selector11/1 -> Product17/3
  Linear Vel Body14/1 -> u Selector11/1
  Sqrt7/1 -> Gain5/1
  Beta_dot/1 -> Divide4/1
  Dot Product7/1 -> Sqrt7/1
  Linear Vel Body13/1 -> Dot Product7/1, Dot Product7/2
  Cyb_dot/1 -> Product16/1
  b3/1 -> Product16/3
  Gain5/1 -> Divide4/2
  Cydelta_T/1 -> Product5/1
  Product8/1 -> Product5/2
  Delta_Thrust/1 -> Product5/3
  Product5/1 -> Integrator20/1
  Cydelta_f/1 -> Product26/1
  Product4/1 -> Product26/2
  Delta_f/1 -> Product26/3
  Product26/1 -> Integrator2/1
  Cydelta_e/1 -> Product28/1
  Product1/1 -> Product28/2
  DeltaElevator/1 -> Product28/3
  Product28/1 -> Integrator1/1
  Cy_ih/1 -> Product3/1
  Product2/1 -> Product3/2
  iH/1 -> Product3/3
  Product3/1 -> Integrator19/1
  q2/1 -> Product35/1
  S2/1 -> Product35/2
  u Selector3/1 -> Product35/3
  Linear Vel Body2/1 -> u Selector3/1
  Cy delta_r/1 -> Product6/1
  Product7/1 -> Product6/2
  DeltaRudder/1 -> Product6/3
  Product6/1 -> Integrator3/1
  q7/1 -> Product7/1
  S7/1 -> Product7/2
  u Selector6/1 -> Product7/3
  Linear Vel Body3/1 -> u Selector6/1
  Integrator3/1 -> Sum1/6
  Integrator1/1 -> Sum1/7
  Integrator19/1 -> Sum1/8
  Integrator2/1 -> Sum1/9
  Integrator20/1 -> Sum1/10
  q1/1 -> Product1/1
  S1/1 -> Product1/2
  u Selector1/1 -> Product1/3
  Linear Vel Body1/1 -> u Selector1/1
  q6/1 -> Product2/1
  S6/1 -> Product2/2
  u Selector4/1 -> Product2/3
  Linear Vel Body4/1 -> u Selector4/1
  q8/1 -> Product4/1
  S8/1 -> Product4/2
  u Selector5/1 -> Product4/3
  Linear Vel Body5/1 -> u Selector5/1
  q9/1 -> Product8/1
  S9/1 -> Product8/2
  u Selector8/1 -> Product8/3
  Linear Vel Body6/1 -> u Selector8/1

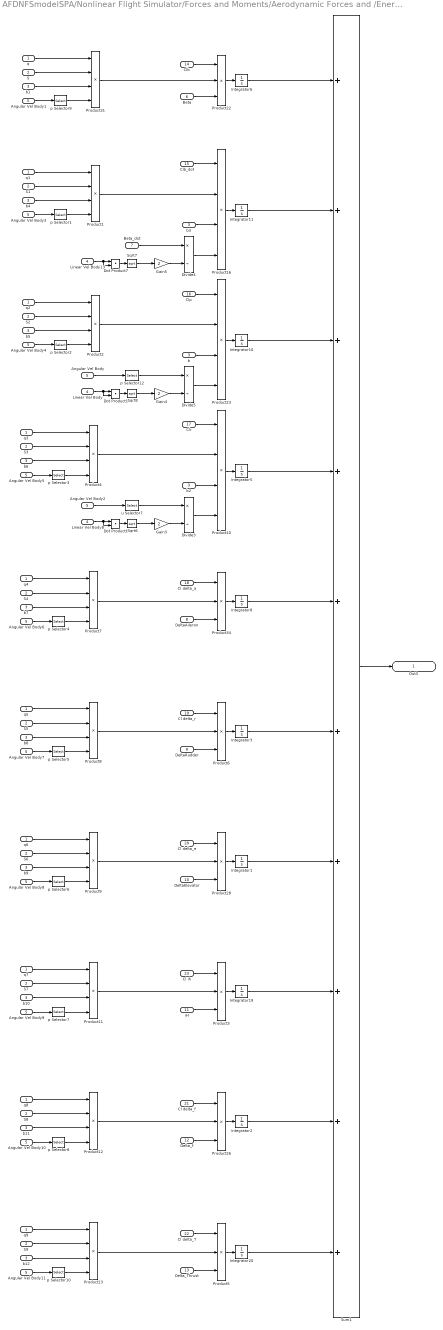
== system AFDNFSmodelSPA/Nonlinear Flight Simulator/Forces and Moments/Aerodynamic Forces and /Energy Analysis1/Lateral-Directional1/L ==
  q : Inport
  S : Inport  Port=2
  b : Inport  Port=3
  Linear Vel Body : Inport  Port=4
  Angular Vel Body : Inport  Port=5
  Beta : Inport  Port=6
  Beta_dot : Inport  Port=7
  DeltaAileron : Inport  Port=8
  DeltaRudder : Inport  Port=9
  DeltaElevator : Inport  Port=10
  iH : Inport  Port=11
  Delta_f : Inport  Port=12
  Delta_Thrust : Inport  Port=13
  Clb : Inport  Port=14
  Clb_dot : Inport  Port=15
  Clp : Inport  Port=16
  Clr : Inport  Port=17
  Cl delta_a : Inport  Port=18
  Cl delta_r : Inport  Port=19
  Cl delta_e : Inport  Port=20
  Cl delta_f : Inport  Port=21
  Cl delta_T : Inport  Port=22
  Cl ih : Inport  Port=23
  Angular Vel Body{1..11} (11 alike) : InportShadow  Port=5
  Divide3 : Product  Inputs=*/
  Divide4 : Product  Inputs=*/
  Divide5 : Product  Inputs=*/
  Dot Product6 : DotProduct  InputSameDT=on  OutDataTypeStr=Inherit: Inherit via internal rule
  Dot Product7 : DotProduct  InputSameDT=on  OutDataTypeStr=Inherit: Inherit via internal rule
  Dot Product9 : DotProduct  InputSameDT=on  OutDataTypeStr=Inherit: Inherit via internal rule
  Gain3 : Gain  Gain=2
  Gain4 : Gain  Gain=2
  Gain5 : Gain  Gain=2
  Integrator{1..3,5..6,8,10..11,19..20} (10 alike) : Integrator
  Linear Vel Body13 : InportShadow  Port=4
  Linear Vel Body8 : InportShadow  Port=4
  Product{1..2,4,7..13,16,23,31} (13 alike) : Product  Inputs=4
  Product{3,5..6,22,26,28,34} (7 alike) : Product  Inputs=3
  S{1..9} (9 alike) : InportShadow  Port=2
  Sqrt6 : Sqrt  SaturateOnIntegerOverflow=on
  Sqrt7 : Sqrt  SaturateOnIntegerOverflow=on
  Sqrt8 : Sqrt  SaturateOnIntegerOverflow=on
  Sum1 : Sum  Inputs=++++++++++
  b{1..12} (12 alike) : InportShadow  Port=3
  p Selector{1..10,12} (11 alike) : Selector  InputPortWidth=3  IndexOptions=Index vector (dialog)  Indices=[1]  OutputSizes=1
  q{1..9} (9 alike) : InportShadow
  u Selector7 : Selector  InputPortWidth=3  IndexOptions=Index vector (dialog)  Indices=[3]  OutputSizes=1
  Out3 : Outport
  wires:
  Integrator11/1 -> Sum1/2
  q/1 -> Product31/1
  S/1 -> Product31/2
  p Selector9/1 -> Product31/4
  Cl delta_a/1 -> Product34/1
  Product7/1 -> Product34/2
  DeltaAileron/1 -> Product34/3
  Product34/1 -> Integrator8/1
  Integrator8/1 -> Sum1/5
  Product2/1 -> Product23/2
  Divide5/1 -> Product23/4
  Product23/1 -> Integrator10/1
  Sqrt8/1 -> Gain4/1
  p Selector12/1 -> Divide5/1
  Dot Product9/1 -> Sqrt8/1
  Linear Vel Body/1 -> Dot Product9/2, Dot Product9/1
  Angular Vel Body/1 -> p Selector12/1
  Clp/1 -> Product23/1
  Sum1/1 -> Out3/1
  Clb/1 -> Product22/1
  Product31/1 -> Product22/2
  Beta/1 -> Product22/3
  Product22/1 -> Integrator6/1
  Integrator6/1 -> Sum1/1
  b/1 -> Product23/3
  Gain4/1 -> Divide5/2
  Product4/1 -> Product10/2
  Divide3/1 -> Product10/4
  Product10/1 -> Integrator5/1
  Sqrt6/1 -> Gain3/1
  u Selector7/1 -> Divide3/1
  Dot Product6/1 -> Sqrt6/1
  Linear Vel Body8/1 -> Dot Product6/1, Dot Product6/2
  Angular Vel Body2/1 -> u Selector7/1
  Clr/1 -> Product10/1
  b2/1 -> Product10/3
  Gain3/1 -> Divide3/2
  Integrator10/1 -> Sum1/3
  Integrator5/1 -> Sum1/4
  Product1/1 -> Product16/2
  Divide4/1 -> Product16/4
  Product16/1 -> Integrator11/1
  Sqrt7/1 -> Gain5/1
  Beta_dot/1 -> Divide4/1
  Dot Product7/1 -> Sqrt7/1
  Linear Vel Body13/1 -> Dot Product7/1, Dot Product7/2
  Clb_dot/1 -> Product16/1
  b3/1 -> Product16/3
  Gain5/1 -> Divide4/2
  Cl delta_T/1 -> Product5/1
  Product13/1 -> Product5/2
  Delta_Thrust/1 -> Product5/3
  Product5/1 -> Integrator20/1
  Cl delta_f/1 -> Product26/1
  Product12/1 -> Product26/2
  Delta_f/1 -> Product26/3
  Product26/1 -> Integrator2/1
  Cl delta_e/1 -> Product28/1
  Product9/1 -> Product28/2
  DeltaElevator/1 -> Product28/3
  Product28/1 -> Integrator1/1
  Cl ih/1 -> Product3/1
  Product11/1 -> Product3/2
  iH/1 -> Product3/3
  Product3/1 -> Integrator19/1
  Cl delta_r/1 -> Product6/1
  Product8/1 -> Product6/2
  DeltaRudder/1 -> Product6/3
  Product6/1 -> Integrator3/1
  Integrator3/1 -> Sum1/6
  Integrator1/1 -> Sum1/7
  Integrator19/1 -> Sum1/8
  Integrator2/1 -> Sum1/9
  Integrator20/1 -> Sum1/10
  Angular Vel Body1/1 -> p Selector9/1
  b1/1 -> Product31/3
  q1/1 -> Product1/1
  S1/1 -> Product1/2
  p Selector1/1 -> Product1/4
  Angular Vel Body3/1 -> p Selector1/1
  b4/1 -> Product1/3
  q2/1 -> Product2/1
  S2/1 -> Product2/2
  p Selector2/1 -> Product2/4
  Angular Vel Body4/1 -> p Selector2/1
  b5/1 -> Product2/3
  q3/1 -> Product4/1
  S3/1 -> Product4/2
  p Selector3/1 -> Product4/4
  Angular Vel Body5/1 -> p Selector3/1
  b6/1 -> Product4/3
  q4/1 -> Product7/1
  S4/1 -> Product7/2
  p Selector4/1 -> Product7/4
  Angular Vel Body6/1 -> p Selector4/1
  b7/1 -> Product7/3
  q5/1 -> Product8/1
  S5/1 -> Product8/2
  p Selector5/1 -> Product8/4
  Angular Vel Body7/1 -> p Selector5/1
  b8/1 -> Product8/3
  q6/1 -> Product9/1
  S6/1 -> Product9/2
  p Selector6/1 -> Product9/4
  Angular Vel Body8/1 -> p Selector6/1
  b9/1 -> Product9/3
  q7/1 -> Product11/1
  S7/1 -> Product11/2
  p Selector7/1 -> Product11/4
  Angular Vel Body9/1 -> p Selector7/1
  b10/1 -> Product11/3
  q8/1 -> Product12/1
  S8/1 -> Product12/2
  p Selector8/1 -> Product12/4
  Angular Vel Body10/1 -> p Selector8/1
  b11/1 -> Product12/3
  q9/1 -> Product13/1
  S9/1 -> Product13/2
  p Selector10/1 -> Product13/4
  Angular Vel Body11/1 -> p Selector10/1
  b12/1 -> Product13/3

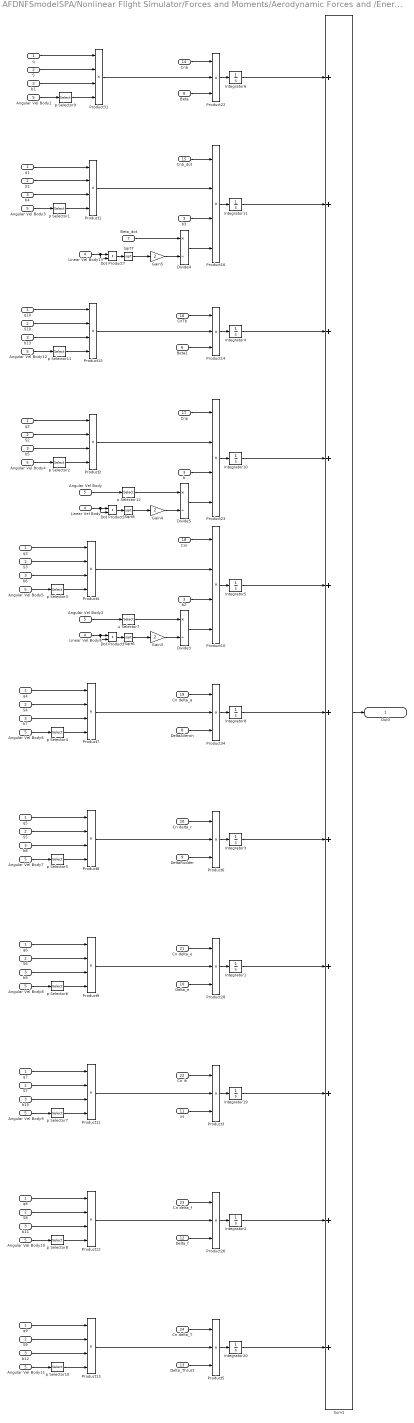
== system AFDNFSmodelSPA/Nonlinear Flight Simulator/Forces and Moments/Aerodynamic Forces and /Energy Analysis1/Lateral-Directional1/N ==
  q : Inport
  S : Inport  Port=2
  b : Inport  Port=3
  Linear Vel Body : Inport  Port=4
  Angular Vel Body : Inport  Port=5
  Beta : Inport  Port=6
  Beta_dot : Inport  Port=7
  DeltaAileron : Inport  Port=8
  DeltaRudder : Inport  Port=9
  Delta_e : Inport  Port=10
  iH : Inport  Port=11
  Delta_f : Inport  Port=12
  Delta_Thrust : Inport  Port=13
  Cnb : Inport  Port=14
  Cnb_dot : Inport  Port=15
  CnTb : Inport  Port=16
  Cnp : Inport  Port=17
  Cnr : Inport  Port=18
  Cn delta_a : Inport  Port=19
  Cn delta_r : Inport  Port=20
  Cn delta_e : Inport  Port=21
  Cn ih : Inport  Port=22
  Cn delta_f : Inport  Port=23
  Cn delta_T : Inport  Port=24
  Angular Vel Body{1..12} (12 alike) : InportShadow  Port=5
  Beta1 : InportShadow  Port=6
  Divide3 : Product  Inputs=*/
  Divide4 : Product  Inputs=*/
  Divide5 : Product  Inputs=*/
  Dot Product6 : DotProduct  InputSameDT=on  OutDataTypeStr=Inherit: Inherit via internal rule
  Dot Product7 : DotProduct  InputSameDT=on  OutDataTypeStr=Inherit: Inherit via internal rule
  Dot Product9 : DotProduct  InputSameDT=on  OutDataTypeStr=Inherit: Inherit via internal rule
  Gain3 : Gain  Gain=2
  Gain4 : Gain  Gain=2
  Gain5 : Gain  Gain=2
  Integrator{1..6,8,10..11,19..20} (11 alike) : Integrator
  Linear Vel Body13 : InportShadow  Port=4
  Linear Vel Body8 : InportShadow  Port=4
  Product{1..2,4,7..13,15..16,23,31} (14 alike) : Product  Inputs=4
  Product{3,5..6,14,22,26,28,34} (8 alike) : Product  Inputs=3
  S{1..10} (10 alike) : InportShadow  Port=2
  Sqrt6 : Sqrt  SaturateOnIntegerOverflow=on
  Sqrt7 : Sqrt  SaturateOnIntegerOverflow=on
  Sqrt8 : Sqrt  SaturateOnIntegerOverflow=on
  Sum1 : Sum  Inputs=+++++++++++
  b{1..13} (13 alike) : InportShadow  Port=3
  p Selector{1..12} (12 alike) : Selector  InputPortWidth=3  IndexOptions=Index vector (dialog)  Indices=[1]  OutputSizes=1
  q{1..10} (10 alike) : InportShadow
  u Selector7 : Selector  InputPortWidth=3  IndexOptions=Index vector (dialog)  Indices=[3]  OutputSizes=1
  Out3 : Outport
  wires:
  Integrator11/1 -> Sum1/2
  q/1 -> Product31/1
  S/1 -> Product31/2
  p Selector9/1 -> Product31/4
  Cn delta_a/1 -> Product34/1
  Product7/1 -> Product34/2
  DeltaAileron/1 -> Product34/3
  Product34/1 -> Integrator8/1
  Product2/1 -> Product23/2
  Divide5/1 -> Product23/4
  Product23/1 -> Integrator10/1
  Sqrt8/1 -> Gain4/1
  p Selector12/1 -> Divide5/1
  Dot Product9/1 -> Sqrt8/1
  Linear Vel Body/1 -> Dot Product9/2, Dot Product9/1
  Angular Vel Body/1 -> p Selector12/1
  Cnp/1 -> Product23/1
  Cnb/1 -> Product22/1
  Product31/1 -> Product22/2
  Beta/1 -> Product22/3
  Product22/1 -> Integrator6/1
  Integrator6/1 -> Sum1/1
  b/1 -> Product23/3
  Gain4/1 -> Divide5/2
  Product4/1 -> Product10/2
  Divide3/1 -> Product10/4
  Product10/1 -> Integrator5/1
  Sqrt6/1 -> Gain3/1
  u Selector7/1 -> Divide3/1
  Dot Product6/1 -> Sqrt6/1
  Linear Vel Body8/1 -> Dot Product6/1, Dot Product6/2
  Angular Vel Body2/1 -> u Selector7/1
  Cnr/1 -> Product10/1
  b2/1 -> Product10/3
  Gain3/1 -> Divide3/2
  Product1/1 -> Product16/2
  Divide4/1 -> Product16/4
  Product16/1 -> Integrator11/1
  Sqrt7/1 -> Gain5/1
  Beta_dot/1 -> Divide4/1
  Dot Product7/1 -> Sqrt7/1
  Linear Vel Body13/1 -> Dot Product7/1, Dot Product7/2
  Cnb_dot/1 -> Product16/1
  b3/1 -> Product16/3
  Gain5/1 -> Divide4/2
  Cn delta_T/1 -> Product5/1
  Product13/1 -> Product5/2
  Delta_Thrust/1 -> Product5/3
  Product5/1 -> Integrator20/1
  Cn delta_f/1 -> Product26/1
  Product12/1 -> Product26/2
  Delta_f/1 -> Product26/3
  Product26/1 -> Integrator2/1
  Cn delta_e/1 -> Product28/1
  Product9/1 -> Product28/2
  Delta_e/1 -> Product28/3
  Product28/1 -> Integrator1/1
  Cn ih/1 -> Product3/1
  Product11/1 -> Product3/2
  iH/1 -> Product3/3
  Product3/1 -> Integrator19/1
  Cn delta_r/1 -> Product6/1
  Product8/1 -> Product6/2
  DeltaRudder/1 -> Product6/3
  Product6/1 -> Integrator3/1
  Angular Vel Body1/1 -> p Selector9/1
  b1/1 -> Product31/3
  q1/1 -> Product1/1
  S1/1 -> Product1/2
  p Selector1/1 -> Product1/4
  Angular Vel Body3/1 -> p Selector1/1
  b4/1 -> Product1/3
  q2/1 -> Product2/1
  S2/1 -> Product2/2
  p Selector2/1 -> Product2/4
  Angular Vel Body4/1 -> p Selector2/1
  b5/1 -> Product2/3
  q3/1 -> Product4/1
  S3/1 -> Product4/2
  p Selector3/1 -> Product4/4
  Angular Vel Body5/1 -> p Selector3/1
  b6/1 -> Product4/3
  q4/1 -> Product7/1
  S4/1 -> Product7/2
  p Selector4/1 -> Product7/4
  Angular Vel Body6/1 -> p Selector4/1
  b7/1 -> Product7/3
  q5/1 -> Product8/1
  S5/1 -> Product8/2
  p Selector5/1 -> Product8/4
  Angular Vel Body7/1 -> p Selector5/1
  b8/1 -> Product8/3
  q6/1 -> Product9/1
  S6/1 -> Product9/2
  p Selector6/1 -> Product9/4
  Angular Vel Body8/1 -> p Selector6/1
  b9/1 -> Product9/3
  q7/1 -> Product11/1
  S7/1 -> Product11/2
  p Selector7/1 -> Product11/4
  Angular Vel Body9/1 -> p Selector7/1
  b10/1 -> Product11/3
  q8/1 -> Product12/1
  S8/1 -> Product12/2
  p Selector8/1 -> Product12/4
  Angular Vel Body10/1 -> p Selector8/1
  b11/1 -> Product12/3
  q9/1 -> Product13/1
  S9/1 -> Product13/2
  p Selector10/1 -> Product13/4
  Angular Vel Body11/1 -> p Selector10/1
  b12/1 -> Product13/3
  q10/1 -> Product15/1
  S10/1 -> Product15/2
  p Selector11/1 -> Product15/4
  CnTb/1 -> Product14/1
  Product15/1 -> Product14/2
  Beta1/1 -> Product14/3
  Product14/1 -> Integrator4/1
  Angular Vel Body12/1 -> p Selector11/1
  b13/1 -> Product15/3
  Integrator20/1 -> Sum1/11
  Integrator2/1 -> Sum1/10
  Integrator19/1 -> Sum1/9
  Integrator1/1 -> Sum1/8
  Integrator3/1 -> Sum1/7
  Integrator8/1 -> Sum1/6
  Integrator5/1 -> Sum1/5
  Integrator10/1 -> Sum1/4
  Integrator4/1 -> Sum1/3
  Sum1/1 -> Out3/1
